simulink model "KF_states_lab"  (R2023b)
settings: Solver=VariableStepAuto  StartTime=0.0  StopTime=100.0  RelTol=1e-3
values from neighbouring files (symbols this model uses):
  A = double(A)    [consistent.m]    (also in dyn_model_mark.m)
  B = double(B)    [consistent.m]    (also in dyn_model_mark.m)
  C = [1 0 0 0 ... (first row only)    [consistent.m]    (also in dyn_model_mark.m)
  D = [0 ... (first row only)    [consistent.m]    (also in dyn_model_mark.m)
  g0 = 9.81    [consistent.m]    (also in dyn_model_mark.m)
  Ip = (mp*Lp^2)/12    (= 3.3282e-05)    [consistent.m]    (also in dyn_model_mark.m = 8.3205e-06)
  Ir = (mr*Lr^2)/12    (= 5.71979166667e-05)    [consistent.m]    (also in dyn_model_mark.m = 1.42994791667e-05)
  Lp = 0.129    [consistent.m]    (also in dyn_model_mark.m = 0.0645)
  Lr = 0.085    [consistent.m]    (also in dyn_model_mark.m)
  mp = 0.024    [consistent.m]    (also in dyn_model_mark.m)
  mr = 0.095    [consistent.m]    (also in dyn_model_mark.m)
  param = [mr mp Lr Lp Ir Ip g0]'    [consistent.m]    (also in dyn_model_mark.m)
  R_tilde = zeros(2,2)    [consistent.m]
undefined symbols (not defined in the file or in its folder): Continuous, rot_pend, Time
libraries: simulink_extras x4, simulink x1, ctrlSharedLib x1
settings Model: Creator=Mark  LastModifiedBy=Mark

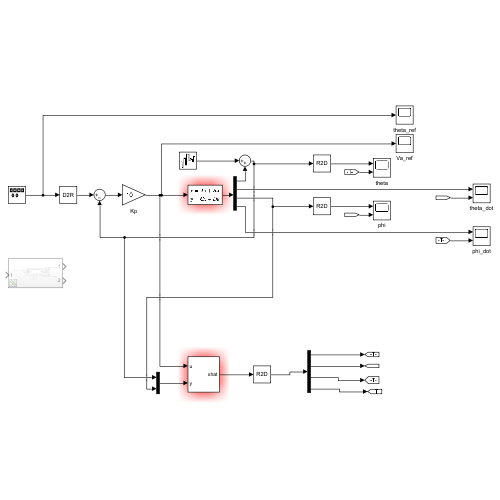
[thumbnail: Simulink's stored preview of the top-level diagram]
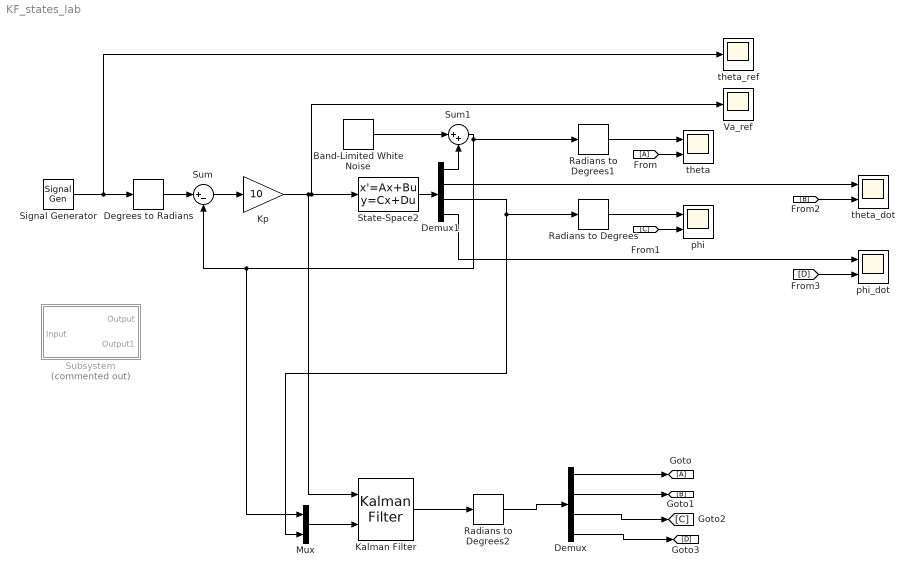
== system KF_states_lab ==
  Band-Limited White Noise : simulink/Sources/Band-Limited White Noise  Cov=[0.1]  Ts=0.1  seed=[23341]
  Degrees to Radians : simulink_extras/Transformations/Degrees to Radians
  Demux : Demux
  Demux1 : Demux
  From : From
  Goto : Goto
  Kalman Filter : ctrlSharedLib/Kalman Filter  TimeDomain=Continuous-Time  UseCurrentEstimator=on  ModelSource=Individual A, B, C, D matrices  ModelSourceVariable=ss(0.95,1,1,0,1)  A=A  B=B  C=C  D=D  NumberOfStates=1  NumberOfInputs=1  NumberOfOutputs=1  InitialEstimateSource=Dialog  X0=0  P0=10  UseK=off  UseGH=off  NumberOfProcessNoiseInputs=1  G=1  TimeInvariantG=on  H=0  TimeInvariantH=on  Q=Q_tilde  TimeInvariantQ=on  R=R_tilde  TimeInvariantR=on  N=0  TimeInvariantN=on  AddInputPort=on  AddEnablePort=off  OutputEstimatedY=off  OutputP=off  Ts=-1
  Kp : Gain  Gain=10
  Mux : Mux  Inputs=2
  Radians to Degrees : simulink_extras/Transformations/Radians to Degrees
  Radians to Degrees1 : simulink_extras/Transformations/Radians to Degrees
  Radians to Degrees2 : simulink_extras/Transformations/Radians to Degrees
  Signal Generator : SignalGenerator  WaveForm=square  Amplitude=5  Frequency=0.05
  State-Space2 : StateSpace  A=A  B=B  C=eye(4)  D=zeros(4,1)  InitialCondition=[0 0 0 0]
  Subsystem : Subsystem  Commented=on
  Sum : Sum  Inputs=|+-
  Sum1 : Sum  Inputs=|++
  Va_ref : Scope
  phi : Scope  NumInputPorts=2
  phi_dot : Scope  NumInputPorts=2
  theta : Scope  NumInputPorts=2
  theta_dot : Scope  NumInputPorts=2
  theta_ref : Scope
  wires:
  Signal Generator/1 -> theta_ref/1, Degrees to Radians/1
  Demux1/3 -> Mux/2, Radians to Degrees/1
  Sum/1 -> Kp/1
  Radians to Degrees1/1 -> theta/1
  Radians to Degrees/1 -> phi/1
  Sum1/1 -> Mux/1, Sum/2, Radians to Degrees1/1
  Kp/1 -> Kalman Filter/1, Va_ref/1, State-Space2/1
  Degrees to Radians/1 -> Sum/1
  Mux/1 -> Kalman Filter/2
  Kalman Filter/1 -> Radians to Degrees2/1
  State-Space2/1 -> Demux1/1
  Demux/1 -> Goto/1
  Demux/2 -> [B]
  Demux/3 -> [C]
  Demux/4 -> [D]
  From/1 -> theta/2
  [C] -> phi/2
  Demux1/2 -> theta_dot/1
  Demux1/4 -> phi_dot/1
  [B] -> theta_dot/2
  [D] -> phi_dot/2
  Radians to Degrees2/1 -> Demux/1
  Band-Limited White Noise/1 -> Sum1/1
  Demux1/1 -> Sum1/2

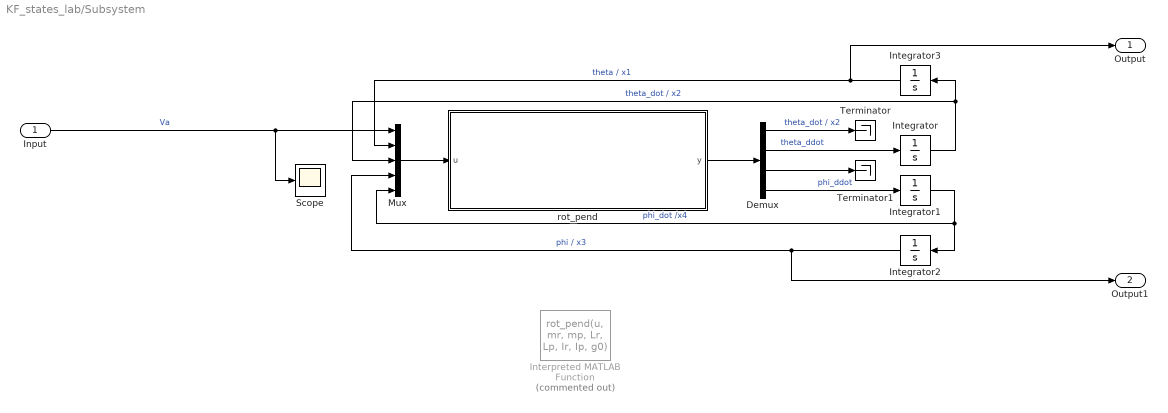
== system KF_states_lab/Subsystem ==
  Input : Inport
  Demux : Demux
  Integrator{,1..3} (4 alike) : Integrator
  Interpreted MATLAB Function : MATLABFcn  Commented=on  MATLABFcn=rot_pend(u, mr, mp, Lr, Lp, Ir, Ip, g0)  OutputDimensions=4  OutputSignalType=real
  Mux : Mux  Inputs=5
  Scope : Scope
  Terminator : Terminator
  Terminator1 : Terminator
  rot_pend : Subsystem
  Output : Outport
  Output1 : Outport  Port=2
  wires:
  Input/1 -> Scope/1, Mux/1  "Va"
  Integrator2/1 -> Output1/1, Mux/4  "phi / x3"
  Integrator/1 -> Integrator3/1, Mux/3  "theta_dot / x2"
  Mux/1 -> rot_pend/1(u)
  rot_pend/1(y) -> Demux/1
  Integrator1/1 -> Mux/5, Integrator2/1  "phi_dot /x4"
  Integrator3/1 -> Mux/2, Output/1  "theta / x1"
  Demux/4 -> Integrator1/1  "phi_ddot"
  Demux/2 -> Integrator/1  "theta_ddot"
  Demux/1 -> Terminator/1  "theta_dot / x2"
  Demux/3 -> Terminator1/1

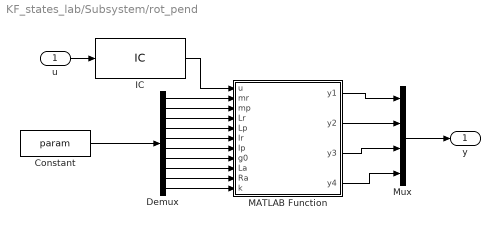
== system KF_states_lab/Subsystem/rot_pend ==
  u : Inport
  Constant : Constant  Value=param  VectorParams1D=off
  Demux : Demux  Outputs=10
  IC : InitialCondition  Value=[0 0 0 pi 0]'
  MATLAB Function : MATLAB Function  TreatAsAtomicUnit=on
  Mux : Mux
  y : Outport
  wires:
  Demux/3 -> MATLAB Function/4(Lr)
  Demux/5 -> MATLAB Function/6(Ir)
  Demux/4 -> MATLAB Function/5(Lp)
  Demux/7 -> MATLAB Function/8(g0)
  Demux/2 -> MATLAB Function/3(mp)
  Demux/6 -> MATLAB Function/7(Ip)
  Demux/1 -> MATLAB Function/2(mr)
  IC/1 -> MATLAB Function/1(u)
  Constant/1 -> Demux/1
  MATLAB Function/1(y1) -> Mux/1
  MATLAB Function/2(y2) -> Mux/2
  MATLAB Function/3(y3) -> Mux/3
  MATLAB Function/4(y4) -> Mux/4
  Mux/1 -> y/1
  Demux/8 -> MATLAB Function/9(La)
  Demux/9 -> MATLAB Function/10(Ra)
  Demux/10 -> MATLAB Function/11(k)
  u/1 -> IC/1

== matlab function KF_states_lab/Subsystem/rot_pend/MATLAB Function ==
  data: u input; y1 output; mr input; mp input; Lr input; Lp input; Ir input; Ip input; g0 input; La input; Ra input; y2 output; y3 output; y4 output; k input
function [y1,y2,y3,y4] = rot_pend(u, mr, mp, Lr, Lp, Ir, Ip, g0,La, Ra, k)
%UNTITLED Summary of this function goes here
%   Detailed explanation goes here
% u(1) = Va
x1 = u(2) ; % theta
x2 = u(3) ; % theta_dot
x3 = u(4) ; % phi
x4 = u(5) ; % phi_dot

H = [(mp*(Lr^2+(Lp^2*(sin(x3))^2)))+4.7912e-05           mp*Lr*Lp*cos(x3);
                     mp*Lr*Lp*cos(x3)                              (mp*Lp^2)+Ip] ;

Q = [mp*Lp^2*sin(x3)*cos(x3)*x4                     (mp*Lp^2*sin(x3)*cos(x3)*x2)-(mp*Lr*Lp*sin(x3)*x4);
     -mp*Lp^2*sin(x3)*cos(x3)*x4                                                   0                                   ] ;

g = [           0     ;
     -mp*g0*Lp*sin(x3)] ;
tau = [((k/Ra)*u(1))-((k^2/Ra)*x2);
                    0                   ] ;

q_ddot = H\[tau - Q*[x2 x4]' - g] ;


y1 = x2 ;
y2 = q_ddot(1) ;
y3 = x4 ;
y4 = q_ddot(2) ;


%Ir+mr*(Lr/2)^2)
